simulink model "Compensated_Model"  (R2024a)
settings: Solver=FixedStepDiscrete  StartTime=0.0  StopTime=20  FixedStep=0.0001  RelTol=1e-3
model workspace (MATLAB code in the model file):
  | Amplitude = 0.35/2;
libraries: simulink x1
settings Model: Creator=Are-Laptop  LastModifiedBy=Are-Laptop
settings ConfigComp: PLC_OutputDir=C:\Users\Are-Laptop\Documents\Skole\PRA-205 - Internship\TwinCAT  PLC_TargetIDE=twincat3  PLC_MultiTBSigbuilderTimeRange=off  PLC_FoldFBCallOutputVar=off  PLC_RemoveUnusedSSMethodCallArguments=off  PLC_UseCallOutputArgSyntax=off  PLC_EnableUnsignedAndDoubleTypes=off  PLC_EnableUDTSplitting=off  PLC_MaxFieldsInUDT=500  PLC_InlineEnumCastFunction=off

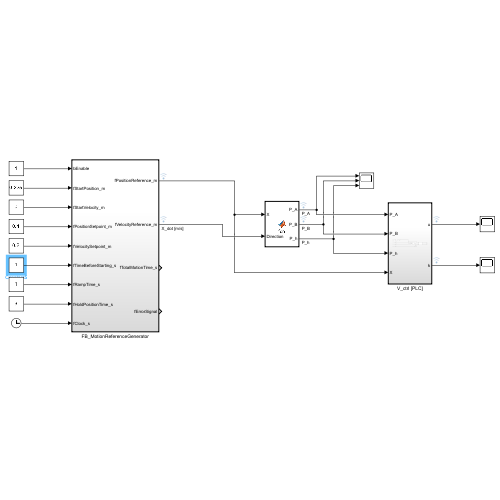
[thumbnail: Simulink's stored preview of the top-level diagram]
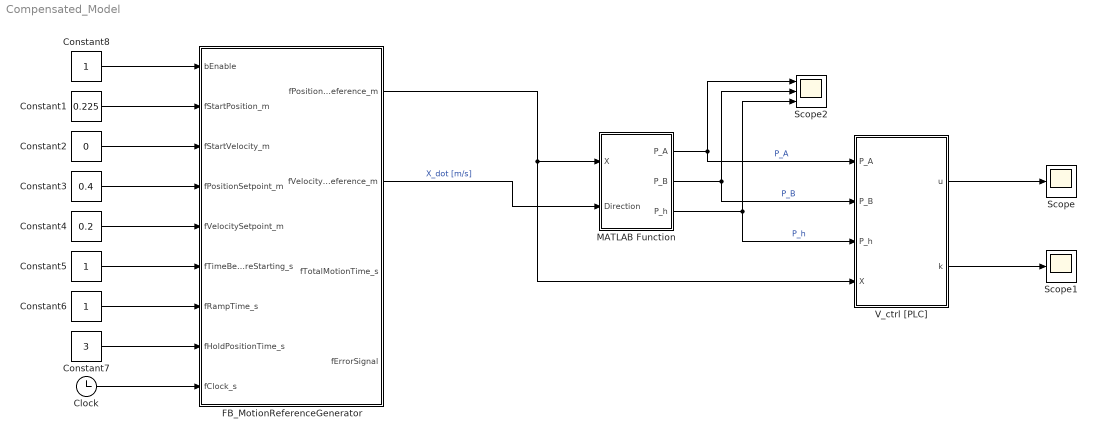
== system Compensated_Model ==
  Clock : Clock
  Constant1 : Constant  Value=0.225
  Constant2 : Constant  Value=0
  Constant3 : Constant  Value=0.4
  Constant4 : Constant  Value=0.2
  Constant5 : Constant
  Constant6 : Constant
  Constant7 : Constant  Value=3
  Constant8 : Constant  OutDataTypeStr=boolean
  FB_MotionReferenceGenerator : Subsystem  TreatAsAtomicUnit=on  VariantControl=Ramp_Profile
  MATLAB Function : MATLAB Function  TreatAsAtomicUnit=on
  Scope : Scope
  Scope1 : Scope
  Scope2 : Scope  NumInputPorts=3
  V_ctrl [PLC] : Subsystem  TreatAsAtomicUnit=on
  wires:
  MATLAB Function/2(P_B) -> Scope2/2, V_ctrl [PLC]/2(P_B)  "P_B"
  MATLAB Function/1(P_A) -> V_ctrl [PLC]/1(P_A), Scope2/1  "P_A"
  FB_MotionReferenceGenerator/2(fVelocityReference_m) -> MATLAB Function/2(Direction)  "X_dot [m/s]"
  V_ctrl [PLC]/1(u) -> Scope/1
  V_ctrl [PLC]/2(k) -> Scope1/1
  Clock/1 -> FB_MotionReferenceGenerator/9(fClock_s)
  Constant1/1 -> FB_MotionReferenceGenerator/2(fStartPosition_m)
  Constant2/1 -> FB_MotionReferenceGenerator/3(fStartVelocity_m)
  Constant3/1 -> FB_MotionReferenceGenerator/4(fPositionSetpoint_m)
  Constant4/1 -> FB_MotionReferenceGenerator/5(fVelocitySetpoint_m)
  Constant5/1 -> FB_MotionReferenceGenerator/6(fTimeBeforeStarting_s)
  Constant6/1 -> FB_MotionReferenceGenerator/7(fRampTime_s)
  Constant7/1 -> FB_MotionReferenceGenerator/8(fHoldPositionTime_s)
  FB_MotionReferenceGenerator/1(fPositionReference_m) -> V_ctrl [PLC]/4(X), MATLAB Function/1(X)
  Constant8/1 -> FB_MotionReferenceGenerator/1(bEnable)
  MATLAB Function/3(P_h) -> Scope2/3, V_ctrl [PLC]/3(P_h)  "P_h"

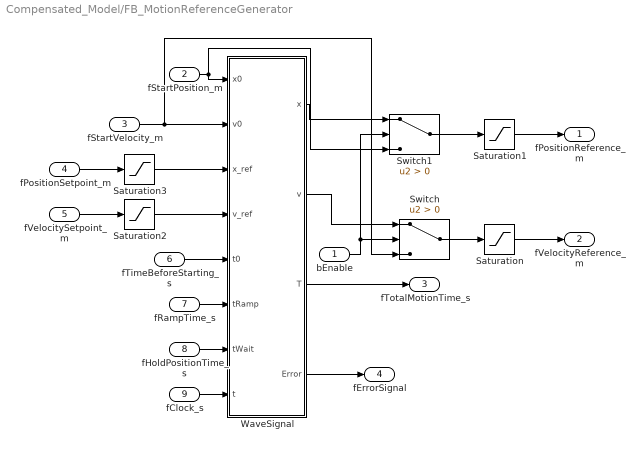
== system Compensated_Model/FB_MotionReferenceGenerator ==
  bEnable : Inport  OutDataTypeStr=boolean
  fStartPosition_m : Inport  Port=2
  fStartVelocity_m : Inport  Port=3
  fPositionSetpoint_m : Inport  Port=4
  fVelocitySetpoint_m : Inport  Port=5
  fTimeBeforeStarting_s : Inport  Port=6
  fRampTime_s : Inport  Port=7
  fHoldPositionTime_s : Inport  Port=8
  fClock_s : Inport  Port=9
  Saturation : Saturate  UpperLimit=0.05  LowerLimit=-0.05
  Saturation1 : Saturate  UpperLimit=0.45  LowerLimit=0
  Saturation2 : Saturate  UpperLimit=0.05  LowerLimit=0
  Saturation3 : Saturate  UpperLimit=0.45  LowerLimit=0
  Switch : Switch  Criteria=u2 > Threshold  SaturateOnIntegerOverflow=off  InputSameDT=off
  Switch1 : Switch  Criteria=u2 > Threshold  SaturateOnIntegerOverflow=off  InputSameDT=off
  WaveSignal : MATLAB Function  TreatAsAtomicUnit=on
  fPositionReference_m : Outport  VectorParamsAs1DForOutWhenUnconnected=off
  fVelocityReference_m : Outport  Port=2  VectorParamsAs1DForOutWhenUnconnected=off
  fTotalMotionTime_s : Outport  Port=3  VectorParamsAs1DForOutWhenUnconnected=off
  fErrorSignal : Outport  Port=4  VectorParamsAs1DForOutWhenUnconnected=off
  wires:
  fClock_s/1 -> WaveSignal/8(t)
  WaveSignal/2(v) -> Switch/1
  Switch/1 -> Saturation/1
  fStartVelocity_m/1 -> Switch/3, WaveSignal/2(v0)
  fTimeBeforeStarting_s/1 -> WaveSignal/5(t0)
  fPositionSetpoint_m/1 -> Saturation3/1
  fHoldPositionTime_s/1 -> WaveSignal/7(tWait)
  fVelocitySetpoint_m/1 -> Saturation2/1
  WaveSignal/1(x) -> Switch1/1
  WaveSignal/3(T) -> fTotalMotionTime_s/1
  fStartPosition_m/1 -> Switch1/3, WaveSignal/1(x0)
  Switch1/1 -> Saturation1/1
  Saturation/1 -> fVelocityReference_m/1
  Saturation2/1 -> WaveSignal/4(v_ref)
  Saturation3/1 -> WaveSignal/3(x_ref)
  fRampTime_s/1 -> WaveSignal/6(tRamp)
  WaveSignal/4(Error) -> fErrorSignal/1
  Saturation1/1 -> fPositionReference_m/1
  bEnable/1 -> Switch1/2, Switch/2

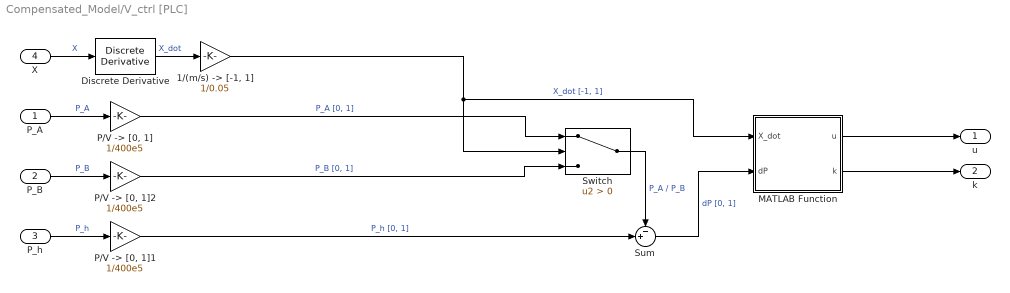
== system Compensated_Model/V_ctrl [PLC] ==
  P_A : Inport
  P_B : Inport  Port=2
  P_h : Inport  Port=3
  X : Inport  Port=4
  "1/(m/s) -> [-1, 1]" : Gain  Gain=1/0.05  OutDataTypeStr=double
  Discrete Derivative : simulink/Quick Insert/Discrete/Discrete Derivative  gainval=1.0  ICPrevScaledInput=0.0  OutMin=[]  OutMax=[]  OutDataType=fixdt(1, 16)  OutScaling=2^-10  DoSatur=off
  MATLAB Function : MATLAB Function  TreatAsAtomicUnit=on
  "P/V -> [0, 1]" : Gain  Gain=1/400e5  OutDataTypeStr=double
  "P/V -> [0, 1]1" : Gain  Gain=1/400e5  OutDataTypeStr=double
  "P/V -> [0, 1]2" : Gain  Gain=1/400e5  OutDataTypeStr=double
  Sum : Sum  Inputs=-+|
  Switch : Switch  Criteria=u2 > Threshold  SaturateOnIntegerOverflow=off  InputSameDT=off
  u : Outport
  k : Outport  Port=2
  wires:
  Sum/1 -> MATLAB Function/2(dP)  "dP [0, 1]"
  Switch/1 -> Sum/1  "P_A / P_B"
  MATLAB Function/1(u) -> u/1
  P_B/1 -> "P/V -> [0, 1]2"/1  "P_B"
  P_A/1 -> "P/V -> [0, 1]"/1  "P_A"
  P_h/1 -> "P/V -> [0, 1]1"/1  "P_h"
  X/1 -> Discrete Derivative/1  "X"
  MATLAB Function/2(k) -> k/1
  "P/V -> [0, 1]"/1 -> Switch/1  "P_A [0, 1]"
  "P/V -> [0, 1]2"/1 -> Switch/3  "P_B [0, 1]"
  "P/V -> [0, 1]1"/1 -> Sum/2  "P_h [0, 1]"
  "1/(m/s) -> [-1, 1]"/1 -> Switch/2, MATLAB Function/1(X_dot)  "X_dot [-1, 1]"
  Discrete Derivative/1 -> "1/(m/s) -> [-1, 1]"/1  "X_dot"

== matlab function Compensated_Model/MATLAB Function ==
  data: X input; Direction input; P_A output; P_B output; P_h output
function [P_A, P_B, P_h] = fcn(X, Direction)

%% fyske_parametere.m
% Constants
L1 = 3.625;
L4 = 0.229;
Lg4x = L1-L4/2;
Lg4y = 0.08157;
abx = 0.550;
aby = -0.130;
g = 9.81;
G1 =100*g;
G4 = (4*76+16)*g;
Cy = -1.055;
Cx = 0.420;
ang_CA = atan2(Cy,Cx);
ang_k = atan2(aby,abx);
b = abs(sqrt(Cy^2+Cx^2));
c = abs(sqrt(abx^2+aby^2));
% Calculations
%syms Ax Ay P gamma beta ang_C ang_AB r_cb r_ab L3 w_A w_C VBx VBy Vp crs_abp
L3 = X + (772+175)/1000;

ang_C = acos((L3^2+b^2-c^2)/(2*L3*b));
beta = ang_CA + pi - ang_C;

bx = L3*cos(beta) + Cx;
by = L3*sin(beta) + Cy;
ang_AB =atan2(by,bx);
gamma = ang_AB + ang_k;

r_cb = [L3*cos(beta);L3*sin(beta);0];
r_ab = [abx*cos(gamma) - aby*sin(gamma); aby*cos(gamma) + abx*sin(gamma); 0 ];
rot_rab = [-1*r_ab(2); r_ab(1)];
rot_rcb = [-1*r_cb(2); r_cb(1)];

crs_abp = cross(r_ab, [cos(beta); sin(beta);0]);
matrix = [1, 0, cos(beta);
    0, 1, sin(beta);
    0, 0, r_ab(1)*sin(beta) - r_ab(2)*cos(beta)];
right = [0;(G1+G4);(G1*cos(gamma)*L1/2+G4*(cos(gamma)*Lg4x-sin(gamma)*Lg4y))];

ANS = inv(matrix)*right;
Ax = ANS(1);
Ay = ANS(2);
P  = ANS(3);

%% pessure_compansetet.m
roh = 850;
u_0 = 0.8/7;
Ffr = 0.05*P;
A = 33.1/100^2;
A2 = 23.6/100^2;
phi = A2/A;
dp0 = 7*10^5;
Pcr = 210*10^5;
Cd = 0.6;

if Direction > 0
    % out stroke
    dp_chk = 4*10^5;
    P3 = dp0;
    P2 = (P/A + phi*P3 + Ffr/A) ;
    P1 = (P2 + dp_chk);

elseif Direction < 0
    % in stroke
    P1 = dp0;
    alpha = 3;
    M =[A, -phi*A;
        1, alpha];
    N =[P-Ffr;
        Pcr+(1+alpha)*P1];
    X = M\N;
    P2 = X(1);
    P3 = X(2);
else
    P1 = 0;
    P3 = 0;
end

P_A = P1;
P_B = P3;
P_h = 180e5;

end

== matlab function Compensated_Model/V_ctrl [PLC]/MATLAB Function ==
  data: X_dot input; dP input; u output; k output
function [u,k] = fcn(X_dot, dP)

phi = 0.7130;
A = 33.1/100^2; % Area
BW = 0.8; % Bandwidth
SpoolTravel = 7; % Maximum Spool Travel
a = (SpoolTravel-BW)/25; % Valve Slope Characteristic [mm/(L/min)]


if X_dot > 0

    Q = X_dot * A; % Wanted Flow

elseif X_dot < 0

    Q = X_dot * (A*phi); % Wanted Flow

else

    Q = 0; % Wanted Flow

end


dP_0 = 7e5/400e5; % Pressure drop with compansator [Pa]
Q_dot = (Q * sqrt(dP_0/dP)) * 6e4; % Referance Flow [L/min]  

u = (Q_dot * a + BW)/SpoolTravel; % Control Signal [-1, 1]
k = Q * 6e4;

end

== matlab function Compensated_Model/FB_MotionReferenceGenerator/WaveSignal ==
  data: x0 input; v0 input; x_ref input; x output; v_ref input; t0 input; tRamp input; tWait input; v output; t input; T output; Error output double
function [x,v,T, Error] = fcn(x0,v0, x_ref,v_ref,t0,tRamp,tWait,t)
x_SP = x_ref - x0;
vs=v_ref;
slopeExt=v0-vs;
slopeRetr=-vs-v0;

as = vs/tRamp;
s_acc=(vs^2-v0^2)/as;

tHold=(x_SP-s_acc)/vs;

if tHold < 0 
Error = 1;
else 
Error = 0;
end

t1=tRamp;
t2=tHold; 
t3=tRamp;
t4=tWait;
t5=t1;
t6=t2;
t7=t3;

x = x0;
x1 = x0 + v0*((t0+t1)-t0)-(slopeExt/t1)*((t0+t1)-t0)^2/2;
x2 = x1 + vs*((t0+t1+t2)-(t0+t1)); 
x4 = x_ref - v0*((t0+t1+t2+t3+t4+t5)-(t0+t1+t2+t3+t4))+(slopeRetr/t5)*((t0+t1+t2+t3+t4+t5)-(t0+t1+t2+t3+t4))^2/2; 
x5 = x4-vs*((t0+t1+t2+t3+t4+t5+t6)-(t0+t1+t2+t3+t4+t5));  

if Error == 1
x = x0;
v = v0; 
elseif t>=0 && t<t0
x = x0; 
v = v0;
elseif t>=t0 && t<(t0+t1)
x = x0 + v0*(t-t0)-(slopeExt/t1)*(t-t0)^2/2;
v = v0-(slopeExt/t1)*(t-t0);  
elseif t>=(t0+t1) && t<(t0+t1+t2)
x = x1 + vs*(t-(t0+t1)); 
v = vs; 
elseif t>=(t0+t1+t2) && t<(t0+t1+t2+t3)
x = x2+vs*(t-(t0+t1+t2))+(slopeExt/t3)*(t-(t0+t1+t2))^2/2; 
v = vs+(slopeExt/t3)*(t-(t0+t1+t2));   
elseif t>=(t0+t1+t2+t3) && t<(t0+t1+t2+t3+t4)
x = x_ref;
v = v0;  
elseif t>=(t0+t1+t2+t3+t4) && t<(t0+t1+t2+t3+t4+t5)
x = x_ref - v0*(t-(t0+t1+t2+t3+t4))+(slopeRetr/t5)*(t-(t0+t1+t2+t3+t4))^2/2; 
v = v0+(slopeRetr/t5)*(t-(t0+t1+t2+t3+t4));     
elseif t>=(t0+t1+t2+t3+t4+t5) && t<(t0+t1+t2+t3+t4+t5+t6)
x = x4-vs*(t-(t0+t1+t2+t3+t4+t5));   
v = -vs;    
elseif t>=(t0+t1+t2+t3+t4+t5+t6) && t<(t0+t1+t2+t3+t4+t5+t6+t7)
x = x5-vs*(t-(t0+t1+t2+t3+t4+t5+t6))-(slopeRetr/t3)*(t-(t0+t1+t2+t3+t4+t5+t6))^2/2;    
v = -vs-(slopeRetr/t3)*(t-(t0+t1+t2+t3+t4+t5+t6));     
else 
x = x0;
v = v0; 
end

T = t0+t1+t2+t3+t4+t5+t6+t7;
